simulink model "power_KundurTwoAreaSystem_1"  (R2021b)
settings: Solver=FixedStepDiscrete  StartTime=0.0  StopTime=30  MaxStep=1/60  RelTol=1e-4
PreLoadFcn:
  | Ts=50e-6;
  | Tctrl=2*Ts;
  | PSSMODEL=1;
undefined symbols (not defined in the file or in its folder): D1, Delta
libraries: spsThreePhaseFaultLib x11, spsGenericPowerSystemStabilizerLib x8, spsThreePhaseBreakerLib x6, spsThreePhaseParallelRLCLoadLib x6, spsThreePhaseVIMeasurementLib x6, spsLoadFlowBusLib x6, spsThreePhasePISectionLineLib x4, spsSynchronousMachinepuStandardLib x4, spsExcitationSystemLib x4, spsSteamTurbineandGovernorLib x4, spsThreePhaseSeriesRLCLoadLib x4, spsThreePhaseTransformerTwoWindingsLib x4
(part 1 of 2)
settings Model: ARTEMISmethode_block_infos=$$__separator__$$  Creator=The MathWorks, Inc.  LastModifiedBy=Pavel
settings SolverCC: AlgebraicLoopSolver=TrustRegion
settings DataIOCC: SaveOutput=off  SignalLogging=off  DSMLogging=off  SaveTime=off  ReturnWorkspaceOutputs=off  TimeSaveName=t  SignalLoggingName=sigsOut
settings OptimizationCC: BlockReduction=off  BooleanDataType=off  OptimizeBlockIOStorage=off  BufferReuse=off  GlobalBufferReuse=off  ExpressionFolding=off  ExpressionDepthLimit=2147483647  LocalBlockOutputs=off  InitFltsAndDblsToZero=on  LifeSpan=inf  OptimizeDataStoreBuffers=off  BusAssignmentInplaceUpdate=off
settings DebuggingCC: SaveWithParameterizedLinksMsg=none  SignalResolutionControl=TryResolveAllWithWarning  MultiTaskDSMMsg=warning  MultiTaskCondExecSysMsg=none  FcnCallInpInsideContextMsg=warning  UnconnectedOutputMsg=none  StateNameClashWarn=warning  SFUnexpectedBacktrackingDiag=warning  SFNoUnconditionalDefaultTransitionDiag=warning  SFExecutionAtInitializationDiag=none  SFMachineParentedDataDiag=warning  ArithmeticOperatorsInVariantConditions=warning
settings HardwareCC: ProdBitPerPointer=32  ProdBitPerSizeT=32  ProdBitPerPtrDiffT=32  ProdLargestAtomicFloat=None  ProdIntDivRoundTo=Undefined  ProdEndianess=Unspecified  ProdWordSize=32  ProdHWDeviceType=32-bit Generic  TargetBitPerPointer=64  TargetBitPerSizeT=64  TargetBitPerPtrDiffT=64  TargetLongLongMode=on  TargetIntDivRoundTo=Zero  TargetEndianess=LittleEndian  TargetWordSize=64  TargetHWDeviceType=MATLAB Host  ProdEqTarget=off
settings ModelReferenceCC: PropagateSignalLabelsOutOfModel=off
settings SFSimCC: SimUseLocalCustomCode=off  CustomCodeUndefinedFunction=UseInterfaceOnly
settings RTWCC: RTWUseLocalCustomCode=off
settings CodeAppCC: StateflowObjectComments=on
settings GRTTargetCC: TargetFcnLib=ansi_tfl_tmw.mat  TargetLangStandard=C89/C90 (ANSI)  CombineOutputUpdateFcns=off  GRTInterface=on
settings ConfigComp: CovMetricSettings=dw  CovSaveCumulativeToWorkspaceVar=on  CovSaveSingleToWorkspaceVar=on  CovExternalEMLEnable=off  CovSFcnEnable=off
settings SimscapeCC: SimscapeNormalizeSystem=off  SimscapeNominalValues={1, 'bar'; 1, 'cm^3/s'; 1, 'bar*kg/s'; 1, 'kJ/kg'; 1, 'kW'; }

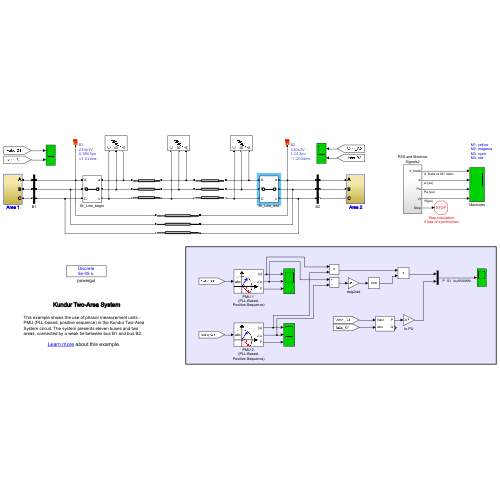
[thumbnail: Simulink's stored preview of the top-level diagram]
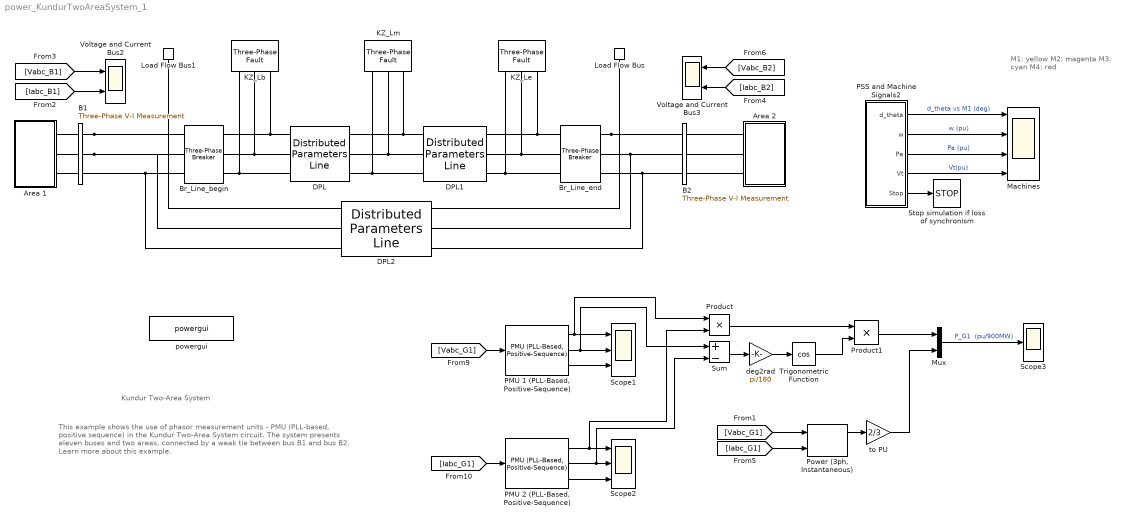
== system power_KundurTwoAreaSystem_1 ==
  note: This example shows the use of phasor measurement units - PMU (PLL-based, positive sequence) in the Kundur Two-Area System circuit. The system presents eleven buses and two areas, connected by a weak tie between bus B1 and bus B2.
      |
      | Learn more about this example.
  note: M1: yellow
      | M2: magenta
      | M3: cyan
      | M4: red
  note: Kundur Two-Area System
  Area 1 : Subsystem
  Area 2 : Subsystem
  B1 : spsThreePhaseVIMeasurementLib/Three-Phase V-I Measurement  VoltageMeasurement=phase-to-ground  SetLabelV=on  LabelV=Vabc_B1  Vpu=on  VpuLL=off  CurrentMeasurement=yes  SetLabelI=on  LabelI=Iabc_B1  Ipu=off  Pbase=100e6  Vbase=230e3  OutputType=Complex  PhasorSimulation=off  PSBequivalent=0
  B2 : spsThreePhaseVIMeasurementLib/Three-Phase V-I Measurement  VoltageMeasurement=phase-to-ground  SetLabelV=on  LabelV=Vabc_B2  Vpu=off  VpuLL=off  CurrentMeasurement=yes  SetLabelI=on  LabelI=Iabc_B2  Ipu=off  Pbase=100e6  Vbase=500e3  OutputType=Complex  PhasorSimulation=off  PSBequivalent=0
  Br_Line_begin : spsThreePhaseBreakerLib/Three-Phase Breaker  InitialState=closed  SwitchA=on  SwitchB=on  SwitchC=on  SwitchTimes=[1 2 3 4 5 6 7 8 9 10 11 12 13 14 15 16 17 18 19 20 21 22 23 24 25]  External=off  BreakerResistance=0.001  SnubberResistance=inf  SnubberCapacitance=0  Measurements=None
      settings: AttributesFormatString=\n
  Br_Line_end : spsThreePhaseBreakerLib/Three-Phase Breaker  InitialState=closed  SwitchA=on  SwitchB=on  SwitchC=on  SwitchTimes=[200]  External=off  BreakerResistance=0.001  SnubberResistance=1e6  SnubberCapacitance=0  Measurements=None
      settings: AttributesFormatString=\n
  DPL : spsDistributedParametersLineLib/Distributed Parameters Line  Phases=3  Length=110  Frequency=60  Resistance=[0.0001*529 1.61]  Inductance=[0.001*529/(377) 0.0061]  Capacitance=[0.00175/529/(377) 5.2489e-9]  x1=[-0.00065 -3.05775777165673e-07 110350.702431426 -199315.843072255;-0.0006 -3.14809127414579e-07 114087.894006705 -197200.498590562;-0.00055 -3.23730627479516e-07 117784.550696487 -195015.089710714;-0.0005 -3.3253710759399e-07 121439.359096251 -192760.392898078;-0.00045 -3.41225438857552e-07 125051.020669976 -190437.209235698;-0.0004 -3.49792534347472e-07 128618.252211502 -188046.364139665;-0.00035 -3.58235350215517e-07 132139.786300449 -185588.707065858;-0.0003 -3.6655088676941e-07 135614.371752522 -183065.111208133;-0.00025 -3.7473618953861e-07 139040.774064055 -180476.473188082;-0.0002 -3.82788350324017e-07 142417.775850622 -177823.712736467;-0.00015 -3.90704508231246e-07 145744.177279569 -175107.772366446;-0.0001 -3.98481850687086e-07 149018.796496306 -172329.617038699;-5e-05 -4.06117614438795e-07 152240.470044219 -169490.233818587]  x2=[-0.00065 -3.14930131728091e-07 73458.8717800933 -217214.376952884;-0.0006 -3.24445421919957e-07 77539.9723093331 -215791.205424005;-0.00055 -3.338454381983e-07 81593.5232556271 -214291.364307353;-0.0005 -3.43126840782096e-07 85618.0844116257 -212715.386489337;-0.00045 -3.52286332033201e-07 89612.2258699133 -211063.831907371;-0.0004 -3.61320657627987e-07 93574.5285310486 -209337.287350933;-0.00035 -3.70226607713589e-07 97503.584607763 -207536.366253084;-0.0003 -3.79001018048348e-07 101397.998125141 -205661.708472514;-0.00025 -3.87640771126053e-07 105256.385416604 -203713.980066206;-0.0002 -3.96142797283573e-07 109077.375615519 -201693.873052788;-0.00015 -4.045040757915e-07 112859.611142262 -199602.105166664;-0.0001 -4.12721635927392e-07 116601.748186561 -197439.419603004;-5e-05 -4.20792558031261e-07 120302.457184942 -195206.584753689]  x3=[-0.00065 -1.54416753788681e-10 -128.79448694137 82.2200529192251;-0.0006 -1.63680232023215e-10 -130.321341891661 79.7777967011709;-0.00055 -1.72885555450693e-10 -131.801894289718 77.3071958118202;-0.0005 -1.82029453463535e-10 -133.235618102324 74.8091280439049;-0.00045 -1.91108677278316e-10 -134.622003934235 72.2844809490081;-0.0004 -2.00120001090046e-10 -135.960559209167 69.7341515222212;-0.00035 -2.09060223218284e-10 -137.250808344805 67.1590458834459;-0.0003 -2.17926167244678e-10 -138.492292921773 64.5600789554538;-0.00025 -2.2671468314153e-10 -139.684571846514 61.9381741388194;-0.0002 -2.35422648390992e-10 -140.827221508002 59.2942629838393;-0.00015 -2.44046969094472e-10 -141.919835928254 56.6292848595577;-0.0001 -2.52584581071892e-10 -142.962026906568 53.9441866200126;-5e-05 -2.61032450950368e-10 -143.953424157453 51.239922267823]  x4=[-0.00065 -2.55233411454253e-10 508.085544669557 -1145.78107221868;-0.0006 -2.62383798237862e-10 529.591487535578 -1136.00084024397;-0.00055 -2.69440961307329e-10 550.90926906779 -1125.81699257992;-0.0005 -2.76402393286219e-10 572.031315159921 -1115.23314749912;-0.00045 -2.83265620810896e-10 592.950121249571 -1104.25306539133;-0.0004 -2.90028205409302e-10 613.658254984543 -1092.88064742744;-0.00035 -2.9668774436733e-10 634.148358863525 -1081.11993417339;-0.0003 -3.03241871582497e-10 654.413152850175 -1068.97510415461;-0.00025 -3.09688258404613e-10 674.445436959683 -1056.45047237138;-0.0002 -3.16024614463136e-10 694.238093816891 -1043.55048876573;-0.00015 -3.22248688480928e-10 713.784091185062 -1030.27973664041;-0.0001 -3.28358269074127e-10 733.076484464402 -1016.64293103046;-5e-05 -3.34351185537842e-10 752.108419159443 -1002.64491702798]  x5=0.000622431770558027  V1=ones(3,3)  V2=ones(3,3)  I1=ones(3,3)  I2=ones(3,3)  nHarmo=1  Measurements=None  Decoupling=off  VsMag0=0  VrMag0=0  VsAngle0=0  VrAngle0=0  IsMag0=0  IrMag0=0  IsAngle0=0  IrAngle0=0
      settings: SourceProductBaseCode=PS
  DPL1 : spsDistributedParametersLineLib/Distributed Parameters Line  Phases=3  Length=110  Frequency=60  Resistance=[0.0001*529 1.61]  Inductance=[0.001*529/(377) 0.0061]  Capacitance=[0.00175/529/(377) 5.2489e-9]  x1=[-0.00065 -3.14930131728091e-07 73458.8717800933 -217214.376952884;-0.0006 -3.24445421919957e-07 77539.9723093331 -215791.205424005;-0.00055 -3.338454381983e-07 81593.5232556271 -214291.364307353;-0.0005 -3.43126840782096e-07 85618.0844116257 -212715.386489337;-0.00045 -3.52286332033201e-07 89612.2258699133 -211063.831907371;-0.0004 -3.61320657627987e-07 93574.5285310486 -209337.287350933;-0.00035 -3.70226607713589e-07 97503.584607763 -207536.366253084;-0.0003 -3.79001018048348e-07 101397.998125141 -205661.708472514;-0.00025 -3.87640771126053e-07 105256.385416604 -203713.980066206;-0.0002 -3.96142797283573e-07 109077.375615519 -201693.873052788;-0.00015 -4.045040757915e-07 112859.611142262 -199602.105166664;-0.0001 -4.12721635927392e-07 116601.748186561 -197439.419603004;-5e-05 -4.20792558031261e-07 120302.457184942 -195206.584753689]  x2=[-0.00065 -3.26364407904076e-07 35485.6832688787 -230363.659450812;-0.0006 -3.35612786810553e-07 39821.3689090633 -229653.8864471;-0.00055 -3.44741924091936e-07 44142.9062064887 -228862.518511059;-0.0005 -3.53748576209219e-07 48448.7597395307 -227989.836811946;-0.00045 -3.62629543141791e-07 52737.3996589316 -227036.151409414;-0.0004 -3.71381669524387e-07 57007.3022313491 -226001.801143346;-0.00035 -3.80001845768179e-07 61256.9503807308 -224887.153513466;-0.0003 -3.88487009165593e-07 65484.8342273244 -223692.604548769;-0.00025 -3.96834144978477e-07 69689.4516241308 -222418.578666815;-0.0002 -4.05040287509224e-07 73869.3086906097 -221065.528522933;-0.00015 -4.13102521154465e-07 78022.9203434482 -219633.934849397;-0.0001 -4.21017981440976e-07 82148.8108242041 -218124.306284621;-5e-05 -4.28783856043408e-07 86245.5142236354 -216537.179192447]  x3=[-0.00065 -2.61540067442109e-10 -144.599429363031 70.9699819573278;-0.0006 -2.7002446451355e-10 -145.91144137221 68.2318277863152;-0.00055 -2.78412923178503e-10 -147.171611741045 65.4694311717841;-0.0005 -2.86702463057546e-10 -148.379492737003 62.683773580098;-0.00045 -2.94890138916633e-10 -149.534655205718 59.8758447421352;-0.0004 -3.02973041713516e-10 -150.636688723465 57.0466423016413;-0.00035 -3.10948299631321e-10 -151.685201742984 54.197171460772;-0.0003 -3.18813079098884e-10 -152.67982173259 51.3284446229489;-0.00025 -3.26564585797509e-10 -153.620195308537 48.4414810331577;-0.0002 -3.34200065653776e-10 -154.505988360572 45.5373064158152;-0.00015 -3.4171680581805e-10 -155.336886170641 42.6169526103345;-0.0001 -3.49112135628341e-10 -156.112593524709 39.681457204517;-5e-05 -3.56383427559182e-10 -156.832834817645 36.7318631659027]  x4=[-0.00065 -1.63989177619071e-10 333.091452979622 -1197.78255581455;-0.0006 -1.72134612436035e-10 355.608619860564 -1191.29145068183;-0.00055 -1.80218888644839e-10 377.999440692142 -1184.37708536917;-0.0005 -1.88239133940642e-10 400.255960122331 -1177.04191651763;-0.00045 -1.96192498768478e-10 422.370270515754 -1169.28855027777;-0.0004 -2.04076157335695e-10 444.334514763229 -1161.1197413837;-0.00035 -2.11887308615944e-10 466.14088907336 -1152.53839217433;-0.0003 -2.19623177344368e-10 487.781645745188 -1143.54755156216;-0.00025 -2.27281015003643e-10 509.249095920913 -1134.15041395007;-0.0002 -2.34858100800513e-10 530.535612317707 -1124.35031809628;-0.00015 -2.42351742632473e-10 551.633631937652 -1114.15074592821;-0.0001 -2.49759278044262e-10 572.535658754838 -1103.55532130526;-5e-05 -2.5707807517382e-10 593.234266378665 -1092.56780873137]  x5=0.000622431770558027  V1=ones(3,3)  V2=ones(3,3)  I1=ones(3,3)  I2=ones(3,3)  nHarmo=1  Measurements=None  Decoupling=off  VsMag0=0  VrMag0=0  VsAngle0=0  VrAngle0=0  IsMag0=0  IrMag0=0  IsAngle0=0  IrAngle0=0
      settings: SourceProductBaseCode=PS
  DPL2 : spsDistributedParametersLineLib/Distributed Parameters Line  Phases=3  Length=220  Frequency=60  Resistance=[0.0001*529 1.61]  Inductance=[0.001*529/(377) 0.0061]  Capacitance=[0.00175/529/(377) 5.2489e-9]  x1=[-0.00125 -1.9006647411866e-07 62839.2443475463 -218987.712338042;-0.0012 -2.00175469260175e-07 66955.6606627248 -217764.389444166;-0.00115 -2.1021334301062e-07 71048.287950487 -216463.695899631;-0.0011 -2.2017652896125e-07 75115.6721198452 -215086.09383466;-0.00105 -2.30061487239536e-07 79156.3680485715 -213632.072704708;-0.001 -2.39864705766871e-07 83168.9400966424 -212102.149116558;-0.00095 -2.49582701506391e-07 87151.9626163157 -210496.866644776;-0.0009 -2.59212021700483e-07 91104.0204586558 -208816.795638581;-0.00085 -2.68749245097534e-07 95023.7094763295 -207062.533019201;-0.0008 -2.78190983167482e-07 98909.6370224928 -205234.702067793;-0.00075 -2.87533881305751e-07 102760.422445592 -203333.952203989;-0.0007 -2.96774620025118e-07 106574.697579902 -201360.958755165;-0.00065 -3.05909916135118e-07 110351.10723163 -199316.4227165;-0.0006 -3.14936523908541e-07 114088.309660409 -197201.070501912;-0.00055 -3.23851236234627e-07 117784.97705601 -195015.653685971;-0.0005 -3.32650885758534e-07 121439.79601011 -192760.948736866;-0.00045 -3.41332346006688e-07 125051.467982937 -190437.756740528;-0.0004 -3.498925324976e-07 128618.709764638 -188046.903116012;-0.00035 -3.5832840383777e-07 132140.253931192 -185589.237322227;-0.0003 -3.66636962802279e-07 135614.849294726 -183065.632556126;-0.00025 -3.74815257399691e-07 139041.261348052 -180476.985442467;-0.0002 -3.82860381920875e-07 142418.272703282 -177824.215715242;-0.00015 -3.90769477971397e-07 145744.683524362 -175108.265890905;-0.0001 -3.98539735487091e-07 149019.311953367 -172330.100933495;-5e-05 -4.06168393732461e-07 152240.994530407 -169490.707911794]  x2=[-0.00125 -2.07645859126878e-07 -17082.1093012616 -232453.302485365;-0.0012 -2.18059622920441e-07 -12697.6983849181 -232733.980459607;-0.00115 -2.28395911168297e-07 -8308.77603679992 -232931.969158782;-0.0011 -2.38651051436448e-07 -3916.90162011914 -233047.198238448;-0.00105 -2.4882140012239e-07 476.364453056495 -233079.626758261;-0.001 -2.58903343749661e-07 4869.46127621022 -233029.243196524;-0.00095 -2.68893300251696e-07 9260.82800295902 -232896.065454275;-0.0009 -2.78787720244519e-07 13648.9044016149 -232680.140848932;-0.00085 -2.8858308828782e-07 18032.1314095277 -232381.54609748;-0.0008 -2.98275924133974e-07 22408.9516870129 -232000.387289211;-0.00075 -3.0786278396456e-07 26777.8101706665 -231536.799848036;-0.0007 -3.17340261613928e-07 31137.1546258722 -230990.948484364;-0.00065 -3.26704989779397e-07 35485.4361983026 -230363.027136587;-0.0006 -3.35953641217643e-07 39821.1099642198 -229653.258902169;-0.00055 -3.45082929926847e-07 44142.6354793796 -228861.895958383;-0.0005 -3.54089612314201e-07 48448.477326344 -227989.219472717;-0.00045 -3.62970488348339e-07 52737.1056600075 -227035.53950297;-0.0004 -3.71722402696293e-07 57006.9967511439 -226001.194887094;-0.00035 -3.8034224584457e-07 61256.6335277802 -224886.553122806;-0.0003 -3.88826955203943e-07 65484.5061142047 -223692.010237017;-0.00025 -3.97173516197577e-07 69689.1123674191 -222417.990645127;-0.0002 -4.05378963332095e-07 73868.9584108423 -221064.94700023;-0.00015 -4.13440381251201e-07 78022.5591650778 -219633.360032291;-0.0001 -4.21354905771493e-07 82148.4388755557 -218123.738377342;-5e-05 -4.29119724900096e-07 86245.1316368605 -216536.61839677]  x3=[-0.00125 -3.080965151432e-11 -106.664284270433 110.129557354209;-0.0012 -3.94517025147854e-11 -108.721104043512 108.099461916423;-0.00115 -4.80797365132012e-11 -110.739295726013 106.030959254546;-0.0011 -5.66906880101712e-11 -112.71814226404 103.924784297725;-0.00105 -6.52814975756306e-11 -114.656940582842 101.781685359894;-0.001 -7.38491129358469e-11 -116.555001836607 99.6024238738994;-0.00095 -8.23904900578784e-11 -118.411651653211 97.3877741209713;-0.0009 -9.09025942311044e-11 -120.226230373812 95.1385229556213;-0.00085 -9.93824011454434e-11 -121.998093287234 92.8554695260786;-0.0008 -1.07826897965877e-10 -123.726610859018 90.5394249903555;-0.00075 -1.16233084402893e-10 -125.411168955104 88.1912122280474;-0.0007 -1.24597973778478e-10 -127.05116906002 85.8116655479677;-0.00065 -1.32918594087269e-10 -128.646028489537 83.4016303917211;-0.0006 -1.41191989052487e-10 -130.195180597696 80.961963033323;-0.00055 -1.49415219176297e-10 -131.698074978128 78.4935302749691;-0.0005 -1.57585362784192e-10 -133.154177659617 75.9972091390648;-0.00045 -1.65699517063052e-10 -134.562971295812 73.473886556623;-0.0004 -1.73754799092496e-10 -135.923955349043 70.9244590521422;-0.00035 -1.81748346869177e-10 -137.236646268157 68.3498324250754;-0.0003 -1.89677320323632e-10 -138.50057766032 65.7509214280037;-0.00025 -1.97538902329347e-10 -139.715300456727 63.1286494416295;-0.0002 -2.05330299703668e-10 -140.880383072153 60.4839481467031;-0.00015 -2.1304874420021e-10 -141.995411558292 57.8177571930017;-0.0001 -2.20691493492394e-10 -143.059989750832 55.1310238654757;-5e-05 -2.28255832147788e-10 -144.073739410211 52.4247027476832]  x4=[-0.00125 -5.16617216311323e-11 55.5524541919917 -1231.05965573251;-0.0012 -5.93136466992287e-11 78.7461313311134 -1229.79381660992;-0.00115 -6.69444979110817e-11 101.911830344732 -1228.0910376001;-0.0011 -7.4551564061591e-11 125.041320570295 -1225.95192369232;-0.00105 -8.21321423963754e-11 148.126384210058 -1223.37723490356;-0.001 -8.96835395720482e-11 171.158819250832 -1220.36788600851;-0.00095 -9.72030726131498e-11 194.130442378119 -1216.92494621447;-0.0009 -1.04688069865396e-10 217.033091883605 -1213.04963878158;-0.00085 -1.12135871944903e-10 239.858630564973 -1208.74334058811;-0.0008 -1.19543832683057e-10 262.598948617016 -1204.00758164131;-0.00075 -1.2690932006668e-10 285.245966513012 -1198.84404453377;-0.0007 -1.34229717173178e-10 307.791637875337 -1193.25456384564;-0.00065 -1.41502423100314e-10 330.227952334312 -1187.2411254928;-0.0006 -1.48724853890304e-10 352.546938374242 -1180.80586602127;-0.00055 -1.55894443447877e-10 374.740666165662 -1173.95107184808;-0.0005 -1.63008644452003e-10 396.801250382764 -1166.67917844897;-0.00045 -1.7006492926094e-10 418.720853005022 -1158.99276949304;-0.0004 -1.77060790810294e-10 440.491686101996 -1150.89457592479;-0.00035 -1.8399374350377e-10 462.106014600351 -1142.38747499383;-0.0003 -1.90861324096287e-10 483.556159032091 -1133.47448923262;-0.00025 -1.97661092569161e-10 504.834498263036 -1124.15878538256;-0.0002 -2.04390632997032e-10 525.933472200577 -1114.44367326887;-0.00015 -2.11047554406229e-10 546.84558447974 -1104.33260462462;-0.0001 -2.17629491624274e-10 567.563405126607 -1093.82917186436;-5e-05 -2.24134106120212e-10 588.079573198153 -1082.93710680773]  x5=0.00124486354111605  V1=ones(3,3)  V2=ones(3,3)  I1=ones(3,3)  I2=ones(3,3)  nHarmo=1  Measurements=None  Decoupling=off  VsMag0=0  VrMag0=0  VsAngle0=0  VrAngle0=0  IsMag0=0  IrMag0=0  IsAngle0=0  IrAngle0=0
      settings: SourceProductBaseCode=PS
  KZ_Lb : spsThreePhaseFaultLib/Three-Phase Fault  InitialStates=0  FaultA=on  FaultB=on  FaultC=on  GroundFault=on  SwitchTimes=[200 200.1]  External=off  SwitchStatus=NaN  FaultResistance=0.001  GroundResistance=0.001  SnubberResistance=1e6  SnubberCapacitance=inf  Measurements=None
  KZ_Le : spsThreePhaseFaultLib/Three-Phase Fault  InitialStates=0  FaultA=on  FaultB=on  FaultC=on  GroundFault=on  SwitchTimes=[200 200.1]  External=off  SwitchStatus=NaN  FaultResistance=0.001  GroundResistance=0.001  SnubberResistance=1e6  SnubberCapacitance=inf  Measurements=None
  KZ_Lm : spsThreePhaseFaultLib/Three-Phase Fault  InitialStates=0  FaultA=on  FaultB=on  FaultC=on  GroundFault=on  SwitchTimes=[200 200.1]  External=off  SwitchStatus=NaN  FaultResistance=0.001  GroundResistance=0.001  SnubberResistance=1e6  SnubberCapacitance=inf  Measurements=None
  Load Flow Bus : spsLoadFlowBusLib/Load Flow Bus  LConnTagsString=a  Phases=single  Connectors=on one side  ID=B2  Vbase=230e3  Vref=1  Vangle=0  VLF=1.013  VLFb=1  VLFc=1  angleLF=-7.203  angleLFb=0  angleLFc=0
      settings: AttributesFormatString=%<ID>\n%<Vbase>V\n%<VLF>pu\n%<angleLF>deg.  SourceProductBaseCode=PS
  Load Flow Bus1 : spsLoadFlowBusLib/Load Flow Bus  LConnTagsString=a  Phases=single  Connectors=on one side  ID=B1  Vbase=230e3  Vref=1  Vangle=0  VLF=0.9905  VLFb=1  VLFc=1  angleLF=13.01  angleLFb=0  angleLFc=0
      settings: AttributesFormatString=%<ID>\n%<Vbase>V\n%<VLF>pu\n%<angleLF>deg.  SourceProductBaseCode=PS
  Machines : Scope  NumInputPorts=4
  Mux : Mux  Inputs=2
  "PMU 1 (PLL-Based, Positive-Sequence)" : spsPMUPLLBasedPositiveSequenceLib/PMU (PLL-Based, Positive-Sequence)  nominalFrequency=60  samplingRate=64  reportingFactor=1
      settings: SourceProductBaseCode=PS
  "PMU 2 (PLL-Based, Positive-Sequence)" : spsPMUPLLBasedPositiveSequenceLib/PMU (PLL-Based, Positive-Sequence)  nominalFrequency=60  samplingRate=64  reportingFactor=1
      settings: SourceProductBaseCode=PS
  PSS and Machine Signals2 : Subsystem
  "Power (3ph, Instantaneous)" : spsPower3phInstantaneousLib/Power (3ph, Instantaneous)
  Product : Product
  Product1 : Product
  Scope1 : Scope  NumInputPorts=3
  Scope2 : Scope  NumInputPorts=3
  Scope3 : Scope
  Stop simulation if loss of synchronism : Stop
  Sum : Sum  Inputs=+-
  Trigonometric Function : Trigonometry  Operator=cos
  Voltage and Current Bus2 : Scope  NumInputPorts=2
  Voltage and Current Bus3 : Scope  NumInputPorts=2
  deg2rad : Gain  Gain=pi/180
  powergui : spspowerguiLib/powergui  Priority=2  SimulationMode=Discrete  SampleTime=Ts  frequency=60  Iterations=50  frequencyindice=60  Pbase=100e6  ErrMax=1e-4  UnitsV=kV  UnitsW=MW  buscounter=0  FunctionMessages=off  echomessages=off  EnableUseOfTLC=off  CurrentSourceSwitches=off  DisableSnubberDevices=off  DisableRonSwitches=off  DisableVfSwitches=off  DisplayEquations=off  AutomaticDiscreteSolvers=off  SolverType=Tustin  Interpol=off  ExternalGateDelay=off  methode=off  Ts=0  x0status=blocks  SPID=off  SwTol=0  HookPort=off  NonlinearTolerance=1e-4  nMaxIteration=100  ContinueOnMaxIteration=off  RestoreLinks=warning  ResistiveCurrentMeasurement=off  Frange=logspace(0,3,50)  Ylog=off  Xlog=off  ShowGrid=off  save=off  variable=ZData  structure=0  ZoomFFT=on  StartTime=0.0  cycles=1  DisplayStyle=1  fundamental=60  FreqAxis=off  MaxFrequency=1000  frequencyindicesteady=1  RmsSteady=1  display=off
  to PU : Gain  Gain=2/3
  wires:
  [Iabc_B1] -> Voltage and Current Bus2/2
  [Vabc_B1] -> Voltage and Current Bus2/1
  [Iabc_B2] -> Voltage and Current Bus3/2
  [Vabc_B2] -> Voltage and Current Bus3/1
  PSS and Machine Signals2/1(d_theta) -> Machines/1  "d_theta vs M1 (deg)"
  PSS and Machine Signals2/2(w) -> Machines/2  "w (pu)"
  PSS and Machine Signals2/3(Pa) -> Machines/3  "Pa (pu)"
  PSS and Machine Signals2/4(Vt) -> Machines/4  "Vt(pu)"
  PSS and Machine Signals2/5(Stop) -> Stop simulation if loss of synchronism/1
  [Iabc_G1] -> "PMU 2 (PLL-Based, Positive-Sequence)"/1
  "PMU 2 (PLL-Based, Positive-Sequence)"/3 -> Scope2/3
  [Vabc_G1] -> "PMU 1 (PLL-Based, Positive-Sequence)"/1
  "PMU 1 (PLL-Based, Positive-Sequence)"/3 -> Scope1/3
  Product/1 -> Product1/1
  [Iabc_G1] -> "Power (3ph, Instantaneous)"/2
  "Power (3ph, Instantaneous)"/1 -> to PU/1
  "PMU 2 (PLL-Based, Positive-Sequence)"/1 -> Product/2, Scope2/1
  [Vabc_G1] -> "Power (3ph, Instantaneous)"/1
  "PMU 2 (PLL-Based, Positive-Sequence)"/2 -> Sum/2, Scope2/2
  deg2rad/1 -> Trigonometric Function/1
  "PMU 1 (PLL-Based, Positive-Sequence)"/1 -> Scope1/1, Product/1
  Trigonometric Function/1 -> Product1/2
  Product1/1 -> Mux/1
  Sum/1 -> deg2rad/1
  to PU/1 -> Mux/2
  "PMU 1 (PLL-Based, Positive-Sequence)"/2 -> Sum/1, Scope1/2
  Mux/1 -> Scope3/1  "P_G1  (pu/900MW)"
  connections:
  Br_Line_end/RConn1 -- DPL2/RConn1 -- B2/LConn1 -- Load Flow Bus/LConn1
  Br_Line_end/RConn2 -- DPL2/RConn2 -- B2/LConn2
  Br_Line_end/RConn3 -- DPL2/RConn3 -- B2/LConn3
  B2/RConn3 -- Area 2/LConn3
  B2/RConn2 -- Area 2/LConn2
  Area 2/LConn1 -- B2/RConn1
  Area 1/RConn3 -- B1/LConn3
  Area 1/RConn2 -- B1/LConn2
  Area 1/RConn1 -- B1/LConn1
  Br_Line_begin/RConn3 -- KZ_Lb/LConn3 -- DPL/LConn3
  Br_Line_begin/RConn2 -- KZ_Lb/LConn2 -- DPL/LConn2
  Br_Line_begin/RConn1 -- KZ_Lb/LConn1 -- DPL/LConn1
  DPL2/LConn3 -- B1/RConn3 -- Br_Line_begin/LConn3
  B1/RConn2 -- DPL2/LConn2 -- Br_Line_begin/LConn2
  B1/RConn1 -- DPL2/LConn1 -- Br_Line_begin/LConn1 -- Load Flow Bus1/LConn1
  DPL1/LConn3 -- DPL/RConn3 -- KZ_Lm/LConn3
  DPL/RConn2 -- KZ_Lm/LConn2 -- DPL1/LConn2
  DPL1/LConn1 -- DPL/RConn1 -- KZ_Lm/LConn1
  DPL1/RConn1 -- KZ_Le/LConn1 -- Br_Line_end/LConn1
  DPL1/RConn2 -- KZ_Le/LConn2 -- Br_Line_end/LConn2
  DPL1/RConn3 -- KZ_Le/LConn3 -- Br_Line_end/LConn3

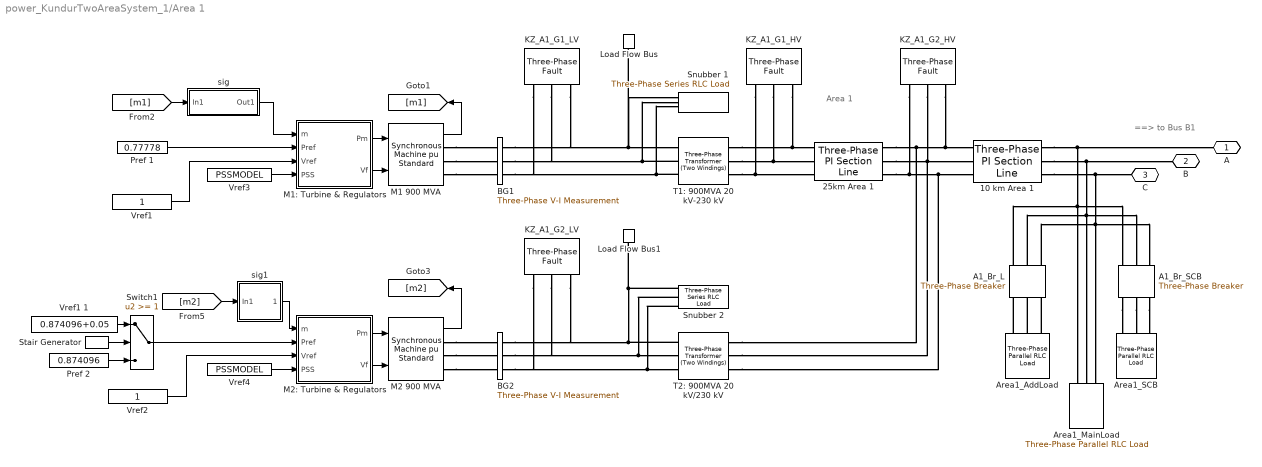
== system power_KundurTwoAreaSystem_1/Area 1 ==
  note: Area 1
  note: ==> to Bus B1
  10 km Area 1 : spsThreePhasePISectionLineLib/Three-Phase PI Section Line  LConnTagsString=a|b|c  RConnTagsString=A|B|C  Length=10  Frequency=60  Resistances=[0.0001*529 1.61]  Inductances=[0.001*529/(377) 0.0061]  Capacitances=[0.00175/529/(377) 5.2489e-9]
  25km Area 1 : spsThreePhasePISectionLineLib/Three-Phase PI Section Line  LConnTagsString=a|b|c  RConnTagsString=A|B|C  Length=25  Frequency=60  Resistances=[0.0001*529 1.61]  Inductances=[0.001*529/(377) 0.0061]  Capacitances=[0.00175/529/(377) 5.2489e-9]
  A1_Br_L : spsThreePhaseBreakerLib/Three-Phase Breaker  InitialState=open  SwitchA=on  SwitchB=on  SwitchC=on  SwitchTimes=[200]  External=off  BreakerResistance=0.001  SnubberResistance=inf  SnubberCapacitance=0  Measurements=None
      settings: AttributesFormatString=\n
  A1_Br_SCB : spsThreePhaseBreakerLib/Three-Phase Breaker  InitialState=closed  SwitchA=off  SwitchB=off  SwitchC=off  SwitchTimes=[200]  External=off  BreakerResistance=0.001  SnubberResistance=inf  SnubberCapacitance=0  Measurements=None
      settings: AttributesFormatString=\n
  Area1_AddLoad : spsThreePhaseParallelRLCLoadLib/Three-Phase Parallel RLC Load  LConnTagsString=A|B|C  Configuration=Y (grounded)  NominalVoltage=230e3  Vabc=[1e3 1e3 1e3]  Vabcp=[1e3 1e3 1e3]  NominalFrequency=60  UnbalancedPower=off  ActivePower=167000000  InductivePower=0  CapacitivePower=87000000  Pabc=[10e3 9e3 11e3]  QLabc=[100 90 110]  QCabc=[100 90 110]  Pabcp=[10e3 9e3 11e3]  QLabcp=[100 90 110]  QCabcp=[100 90 110]  Measurements=None  LoadType=constant Z
  Area1_MainLoad : spsThreePhaseParallelRLCLoadLib/Three-Phase Parallel RLC Load  LConnTagsString=A|B|C  Configuration=Y (grounded)  NominalVoltage=230e3  Vabc=[1e3 1e3 1e3]  Vabcp=[1e3 1e3 1e3]  NominalFrequency=60  UnbalancedPower=off  ActivePower=1190000000  InductivePower=0  CapacitivePower=87000000  Pabc=[10e3 9e3 11e3]  QLabc=[100 90 110]  QCabc=[100 90 110]  Pabcp=[10e3 9e3 11e3]  QLabcp=[100 90 110]  QCabcp=[100 90 110]  Measurements=None  LoadType=constant Z
  Area1_SCB : spsThreePhaseParallelRLCLoadLib/Three-Phase Parallel RLC Load  LConnTagsString=A|B|C  Configuration=Y (grounded)  NominalVoltage=230e3  Vabc=[1e3 1e3 1e3]  Vabcp=[1e3 1e3 1e3]  NominalFrequency=60  UnbalancedPower=off  ActivePower=0  InductivePower=0  CapacitivePower=200000000  Pabc=[10e3 9e3 11e3]  QLabc=[100 90 110]  QCabc=[100 90 110]  Pabcp=[10e3 9e3 11e3]  QLabcp=[100 90 110]  QCabcp=[100 90 110]  Measurements=None  LoadType=constant Z
  BG1 : spsThreePhaseVIMeasurementLib/Three-Phase V-I Measurement  VoltageMeasurement=phase-to-ground  SetLabelV=on  LabelV=Vabc_G1  Vpu=on  VpuLL=off  CurrentMeasurement=yes  SetLabelI=on  LabelI=Iabc_G1  Ipu=on  Pbase=900e6  Vbase=20e3  OutputType=Complex  PhasorSimulation=off  PSBequivalent=0
  BG2 : spsThreePhaseVIMeasurementLib/Three-Phase V-I Measurement  VoltageMeasurement=no  SetLabelV=on  LabelV=Vabc_G2  Vpu=on  VpuLL=off  CurrentMeasurement=no  SetLabelI=on  LabelI=Iabc_G2  Ipu=on  Pbase=900e6  Vbase=20e3  OutputType=Complex  PhasorSimulation=off  PSBequivalent=0
  KZ_A1_G1_HV : spsThreePhaseFaultLib/Three-Phase Fault  InitialStates=0  FaultA=on  FaultB=on  FaultC=on  GroundFault=on  SwitchTimes=[200 200.1]  External=off  SwitchStatus=NaN  FaultResistance=0.001  GroundResistance=0.001  SnubberResistance=1e6  SnubberCapacitance=inf  Measurements=None
  KZ_A1_G1_LV : spsThreePhaseFaultLib/Three-Phase Fault  InitialStates=0  FaultA=off  FaultB=on  FaultC=on  GroundFault=on  SwitchTimes=[200 200.1]  External=off  SwitchStatus=NaN  FaultResistance=0.001  GroundResistance=0.001  SnubberResistance=1e6  SnubberCapacitance=inf  Measurements=None
  KZ_A1_G2_HV : spsThreePhaseFaultLib/Three-Phase Fault  InitialStates=0  FaultA=on  FaultB=on  FaultC=on  GroundFault=on  SwitchTimes=[200 200.1]  External=off  SwitchStatus=NaN  FaultResistance=0.001  GroundResistance=0.001  SnubberResistance=1e6  SnubberCapacitance=inf  Measurements=None
  KZ_A1_G2_LV : spsThreePhaseFaultLib/Three-Phase Fault  InitialStates=0  FaultA=on  FaultB=on  FaultC=on  GroundFault=on  SwitchTimes=[200 200.1]  External=off  SwitchStatus=NaN  FaultResistance=0.001  GroundResistance=0.001  SnubberResistance=1e6  SnubberCapacitance=inf  Measurements=None
  Load Flow Bus : spsLoadFlowBusLib/Load Flow Bus  LConnTagsString=a  Phases=single  Connectors=on one side  ID=M1_Area1  Vbase=20e3  Vref=1  Vangle=0  VLF=1  VLFb=1  VLFc=1  angleLF=8.951  angleLFb=0  angleLFc=0
      settings: AttributesFormatString=%<ID>\n%<Vbase>V\n%<VLF>pu\n%<angleLF>deg.  SourceProductBaseCode=PS
  Load Flow Bus1 : spsLoadFlowBusLib/Load Flow Bus  LConnTagsString=a  Phases=single  Connectors=on one side  ID=M2_Area1  Vbase=20e3  Vref=1  Vangle=0  VLF=1  VLFb=1  VLFc=1  angleLF=0  angleLFb=0  angleLFc=0
      settings: AttributesFormatString=%<ID>\n%<Vbase>V\n%<VLF>pu\n%<angleLF>deg.  SourceProductBaseCode=PS
  M1 900 MVA : spsSynchronousMachinepuStandardLib/Synchronous Machine pu Standard  PresetModel=No  MechanicalLoad=Mechanical power Pm  ShowDetailedParameters=on  RotorType=Round  Units=per unit standard parameters  MeasurementBus=off  NominalParameters="[900E6  20000   60 ]"  Reactances1=[1.8 .3 .25 1.7 .55 .25 .2]  Reactances2=[ 1.305, 0.296, 0.252, 0.474, 0.243, 0.18 ]  dAxisTimeConstants=Open-circuit  qAxisTimeConstants=Open-circuit  TimeConstants1=[]  TimeConstants2=[8 .03 .4 .05]  TimeConstants3=[]  TimeConstants4=[]  TimeConstants5=[ 1.01, 0.053, 0.1 ]  TimeConstants6=[]  TimeConstants7=[]  TimeConstants8=[]  StatorResistance=0.0025  Mechanical="[ 6.5 0  4]"  PolePairs=4  InitialConditions=[0 -32.4356 0.783664 0.783664 0.783664 1.92383 -118.076 121.924 1.8267]  SetSaturation=off  Saturation=[0.6404,0.7127,0.8441,0.9214,0.9956,1.082,1.19,1.316,1.457;0.7,0.7698,0.8872,0.9466,0.9969,1.046,1.1,1.151,1.201]  LoadFlowParameters=[1 700000000 0 0 0]  TsPowergui=0  TsBlock=-1  IterativeModel=Trapezoidal non iterative  IterativeDiscreteModel=Trapezoidal non iterative  BusType=PV  Pref=700000000  Qref=0  Qmin=-Inf  Qmax=Inf  PLF=0  QLF=0
      settings: SourceProductBaseCode=PS
  M1: Turbine & Regulators : Subsystem
  M2 900 MVA : spsSynchronousMachinepuStandardLib/Synchronous Machine pu Standard  PresetModel=No  MechanicalLoad=Mechanical power Pm  ShowDetailedParameters=on  RotorType=Round  Units=per unit standard parameters  MeasurementBus=off  NominalParameters="[900E6  20000   60 ]"  Reactances1=[1.8 .3 .25 1.7 .55 .25 .2]  Reactances2=[ 1.305, 0.296, 0.252, 0.474, 0.243, 0.18 ]  dAxisTimeConstants=Open-circuit  qAxisTimeConstants=Open-circuit  TimeConstants1=[]  TimeConstants2=[8 .03 .4 .05]  TimeConstants3=[]  TimeConstants4=[]  TimeConstants5=[ 1.01, 0.053, 0.1 ]  TimeConstants6=[]  TimeConstants7=[]  TimeConstants8=[]  StatorResistance=0.0025  Mechanical="[ 6.5 0  4]"  PolePairs=4  InitialConditions=[0 -38.7801 0.934029 0.934029 0.934029 -9.29278 -129.293 110.707 2.09095]  SetSaturation=off  Saturation=[0.6404,0.7127,0.8441,0.9214,0.9956,1.082,1.19,1.316,1.457;0.7,0.7698,0.8872,0.9466,0.9969,1.046,1.1,1.151,1.201]  LoadFlowParameters=[2 700000000 0 0 0]  TsPowergui=0  TsBlock=-1  IterativeModel=Trapezoidal non iterative  IterativeDiscreteModel=Trapezoidal non iterative  BusType=swing  Pref=0  Qref=0  Qmin=-Inf  Qmax=Inf  PLF=0  QLF=0
      settings: SourceProductBaseCode=PS
  M2: Turbine & Regulators : Subsystem
  Pref 1 : Constant  Value=0.77778
  Pref 2 : Constant  Value=0.874096
  Snubber 1 : spsThreePhaseSeriesRLCLoadLib/Three-Phase Series RLC Load  LConnTagsString=A|B|C  Configuration=Y (grounded)  NominalVoltage=20000  Vabc=[1e3 1e3 1e3]  Vabcp=[1e3 1e3 1e3]  NominalFrequency=60  UnbalancedPower=off  ActivePower=1000000  InductivePower=0  CapacitivePower=10000000  Pabc=[10e3 9e3 11e3]  QLabc=[100 90 110]  QCabc=[100 90 110]  Pabcp=[10e3 9e3 11e3]  QLabcp=[100 90 110]  QCabcp=[100 90 110]  Measurements=None  LoadType=constant Z
  Snubber 2 : spsThreePhaseSeriesRLCLoadLib/Three-Phase Series RLC Load  LConnTagsString=A|B|C  Configuration=Y (grounded)  NominalVoltage=20000  Vabc=[1e3 1e3 1e3]  Vabcp=[1e3 1e3 1e3]  NominalFrequency=60  UnbalancedPower=off  ActivePower=1000000  InductivePower=0  CapacitivePower=10000000  Pabc=[10e3 9e3 11e3]  QLabc=[100 90 110]  QCabc=[100 90 110]  Pabcp=[10e3 9e3 11e3]  QLabcp=[100 90 110]  QCabcp=[100 90 110]  Measurements=None  LoadType=constant Z
  Stair Generator : spsStairGeneratorLib/Stair Generator  t=[0 15 20]  e=[0 1 0 ]  Ts=0
  Switch1 : Switch  Threshold=1  InputSameDT=on
  T1: 900MVA 20 kV-230 kV : spsThreePhaseTransformerTwoWindingsLib/Three-Phase Transformer (Two Windings)  Winding1Connection=Delta (D1)  Winding2Connection=Yg  CoreType=Three single-phase transformers  SetSaturation=off  Hysteresis=off  DataFile='hysteresis'  SetInitialFlux=off  Measurements=None  UNITS=pu  NominalPower="[ 900e6   60 ]"  Winding1="[ 20e3  1e-6   0  ]"  Winding2="[ 230e3  1e-6   0.15 ]"  Rm=500  Lm=500  L0=0.5  Saturation="[ 0,0  ;  0.005,1.2  ;  1.0,1.4 ]"  InitialFluxes=[ 0.8 , -0.8 , 0.7 ]  BreakLoop=off  DiscreteSolver=Trapezoidal iterative  DataType=off  TransfoNumber=0
  T2: 900MVA 20 kV/230 kV : spsThreePhaseTransformerTwoWindingsLib/Three-Phase Transformer (Two Windings)  Winding1Connection=Delta (D1)  Winding2Connection=Yg  CoreType=Three single-phase transformers  SetSaturation=off  Hysteresis=off  DataFile='hysteresis'  SetInitialFlux=off  Measurements=None  UNITS=pu  NominalPower=[ 900e6 60 ]  Winding1="[ 20e3 1e-6  0.0]"  Winding2=[ 230e3 1e-6 0.15]  Rm=500  Lm=500  L0=0.5  Saturation="[ 0,0  ;  0.005,1.2  ;  1.0,1.4 ]"  InitialFluxes=[ 0.8 , -0.8 , 0.7 ]  BreakLoop=off  DiscreteSolver=Trapezoidal iterative  DataType=off  TransfoNumber=0
  Vref1 : Constant
  Vref1 1 : Constant  Value=0.874096+0.05
  Vref2 : Constant
  Vref3 : Constant  Value=PSSMODEL
  Vref4 : Constant  Value=PSSMODEL
  sig : Subsystem
  sig1 : Subsystem
  " A" : PMIOPort  Side=Right
  " B" : PMIOPort  Port=2  Side=Right
  " C" : PMIOPort  Port=3  Side=Right
  wires:
  Pref 1/1 -> M1: Turbine & Regulators/2(Pref)
  Vref2/1 -> M2: Turbine & Regulators/3(Vref)
  Vref4/1 -> M2: Turbine & Regulators/4(PSS)
  sig/1(Out1) -> M1: Turbine & Regulators/1(m)
  M1 900 MVA/1 -> [m1]
  M2 900 MVA/1 -> [m2]
  [m1] -> sig/1(In1)
  Vref3/1 -> M1: Turbine & Regulators/4(PSS)
  sig1/1(Out1) -> M2: Turbine & Regulators/1(m)
  [m2] -> sig1/1(In1)
  Stair Generator/1 -> Switch1/2
  Pref 2/1 -> Switch1/3
  Vref1 1/1 -> Switch1/1
  Switch1/1 -> M2: Turbine & Regulators/2(Pref)
  Vref1/1 -> M1: Turbine & Regulators/3(Vref)
  M1: Turbine & Regulators/1(Pm) -> M1 900 MVA/1
  M1: Turbine & Regulators/2(Vf) -> M1 900 MVA/2
  M2: Turbine & Regulators/2(Vf) -> M2 900 MVA/2
  M2: Turbine & Regulators/1(Pm) -> M2 900 MVA/1
  connections:
  T1: 900MVA 20 kV-230 kV/RConn1 -- KZ_A1_G1_HV/LConn1 -- 25km Area 1/LConn1
  T1: 900MVA 20 kV-230 kV/RConn2 -- KZ_A1_G1_HV/LConn2 -- 25km Area 1/LConn2
  Snubber 2/LConn1 -- KZ_A1_G2_LV/LConn1 -- BG2/RConn1 -- T2: 900MVA 20 kV/230 kV/LConn1 -- Load Flow Bus1/LConn1
  Snubber 2/LConn2 -- KZ_A1_G2_LV/LConn2 -- BG2/RConn2 -- T2: 900MVA 20 kV/230 kV/LConn2
  Snubber 2/LConn3 -- KZ_A1_G2_LV/LConn3 -- BG2/RConn3 -- T2: 900MVA 20 kV/230 kV/LConn3
  T1: 900MVA 20 kV-230 kV/RConn3 -- KZ_A1_G1_HV/LConn3 -- 25km Area 1/LConn3
  10 km Area 1/RConn1 -- " A"/RConn1 -- A1_Br_L/RConn1 -- A1_Br_SCB/RConn1 -- Area1_MainLoad/LConn1
  10 km Area 1/RConn2 -- " B"/RConn1 -- A1_Br_L/RConn2 -- A1_Br_SCB/RConn2 -- Area1_MainLoad/LConn2
  10 km Area 1/RConn3 -- " C"/RConn1 -- A1_Br_L/RConn3 -- A1_Br_SCB/RConn3 -- Area1_MainLoad/LConn3
  Snubber 1/LConn1 -- Load Flow Bus/LConn1 -- BG1/RConn1 -- KZ_A1_G1_LV/LConn1 -- T1: 900MVA 20 kV-230 kV/LConn1
  T1: 900MVA 20 kV-230 kV/LConn2 -- BG1/RConn2 -- KZ_A1_G1_LV/LConn2 -- Snubber 1/LConn2
  T1: 900MVA 20 kV-230 kV/LConn3 -- BG1/RConn3 -- KZ_A1_G1_LV/LConn3 -- Snubber 1/LConn3
  25km Area 1/RConn2 -- KZ_A1_G2_HV/LConn2 -- 10 km Area 1/LConn2 -- T2: 900MVA 20 kV/230 kV/RConn2
  25km Area 1/RConn1 -- T2: 900MVA 20 kV/230 kV/RConn1 -- KZ_A1_G2_HV/LConn1 -- 10 km Area 1/LConn1
  25km Area 1/RConn3 -- KZ_A1_G2_HV/LConn3 -- 10 km Area 1/LConn3 -- T2: 900MVA 20 kV/230 kV/RConn3
  M1 900 MVA/RConn1 -- BG1/LConn1
  M1 900 MVA/RConn2 -- BG1/LConn2
  M1 900 MVA/RConn3 -- BG1/LConn3
  M2 900 MVA/RConn1 -- BG2/LConn1
  M2 900 MVA/RConn2 -- BG2/LConn2
  M2 900 MVA/RConn3 -- BG2/LConn3
  A1_Br_SCB/LConn1 -- Area1_SCB/LConn1
  A1_Br_SCB/LConn2 -- Area1_SCB/LConn2
  A1_Br_SCB/LConn3 -- Area1_SCB/LConn3
  Area1_AddLoad/LConn2 -- A1_Br_L/LConn2
  Area1_AddLoad/LConn1 -- A1_Br_L/LConn1
  Area1_AddLoad/LConn3 -- A1_Br_L/LConn3
